simulink model "MBD_week2_prob4"  (R2020b)
settings: Solver=VariableStepAuto  StartTime=0.0  StopTime=0.2  RelTol=1e-3
model workspace (MAT data in the model file):
  J = Simulink.Parameter
  J.Value = 3.2284e-06
  J.DataType = 'auto'
  J.Dimensions = [1 1]
  Ke = Simulink.Parameter
  Ke.Value = 0.0274
  Ke.DataType = 'auto'
  Ke.Dimensions = [1 1]
  Kt = Simulink.Parameter
  Kt.Value = 0.0274
  Kt.DataType = 'auto'
  Kt.Dimensions = [1 1]
  L = Simulink.Parameter
  L.Value = 2.75e-06
  L.DataType = 'auto'
  L.Dimensions = [1 1]
  R = Simulink.Parameter
  R.Value = 4
  R.DataType = 'auto'
  R.Dimensions = [1 1]
  Ts = Simulink.Parameter
  Ts.Value = 0.01
  Ts.DataType = 'auto'
  Ts.Dimensions = [1 1]
  b = Simulink.Parameter
  b.Value = 3.5077e-06
  b.DataType = 'auto'
  b.Dimensions = [1 1]
  kd = Simulink.Parameter
  kd.Value = 50
  kd.DataType = 'auto'
  kd.Dimensions = [1 1]
  ki = Simulink.Parameter
  ki.Value = 22000
  ki.DataType = 'auto'
  ki.Dimensions = [1 1]
  kp = Simulink.Parameter
  kp.Value = 22000
  kp.DataType = 'auto'
  kp.Dimensions = [1 1]
settings Model: Creator=varunraj  LastModifiedBy=varunraj

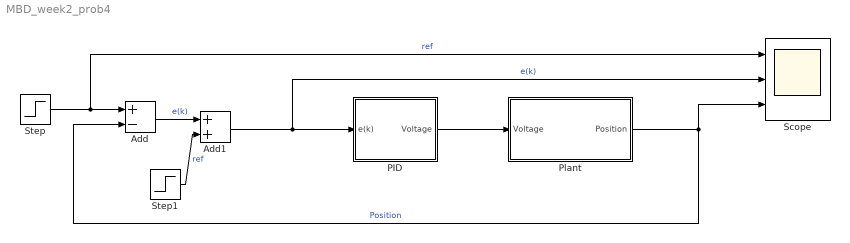
== system MBD_week2_prob4 ==
  Add : Sum  Inputs=+-
  Add1 : Sum
  PID : Subsystem  TreatAsAtomicUnit=on
  Plant : Subsystem  TreatAsAtomicUnit=on
  Scope : Scope  NumInputPorts=3
  Step : Step  Time=0.01  SampleTime=0
  Step1 : Step  Time=0.01  SampleTime=0
  wires:
  Step/1 -> Scope/1, Add/1  "ref"
  Add/1 -> Add1/1  "e(k)"
  Step1/1 -> Add1/2  "ref"
  Add1/1 -> Scope/2, PID/1(e(k))  "e(k)"
  PID/1(Voltage) -> Plant/1(Voltage)
  Plant/1(Position) -> Add/2, Scope/3  "Position"

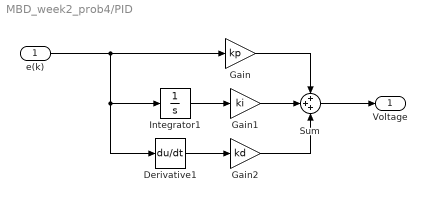
== system MBD_week2_prob4/PID ==
  e(k) : Inport  OutDataTypeStr=double  PortDimensions=1  SampleTime=0
  Derivative1 : Derivative
  Gain : Gain  Gain=kp
  Gain1 : Gain  Gain=ki
  Gain2 : Gain  Gain=kd
  Integrator1 : Integrator
  Sum : Sum  Inputs=+++
  Voltage : Outport  OutDataTypeStr=double  PortDimensions=1  SampleTime=0
  wires:
  Gain/1 -> Sum/1
  Sum/1 -> Voltage/1
  Derivative1/1 -> Gain2/1
  Gain2/1 -> Sum/3
  e(k)/1 -> Gain/1, Integrator1/1, Derivative1/1
  Gain1/1 -> Sum/2
  Integrator1/1 -> Gain1/1

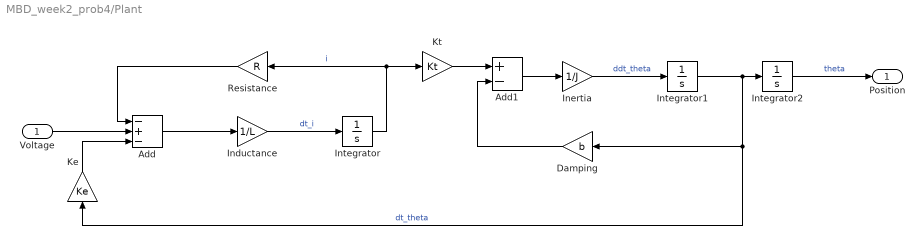
== system MBD_week2_prob4/Plant ==
  Voltage : Inport
  Add : Sum  Inputs=-+-
  Add1 : Sum  Inputs=+-
  Damping : Gain  Gain=b
  Inductance : Gain  Gain=1/L
  Inertia : Gain  Gain=1/J
  Integrator : Integrator
  Integrator1 : Integrator
  Integrator2 : Integrator
  Ke : Gain  Gain=Ke
  Kt : Gain  Gain=Kt
  Resistance : Gain  Gain=R
  Position : Outport
  wires:
  Add/1 -> Inductance/1
  Voltage/1 -> Add/2
  Kt/1 -> Add1/1
  Integrator1/1 -> Ke/1, Damping/1, Integrator2/1  "dt_theta"
  Integrator/1 -> Resistance/1, Kt/1  "i"
  Ke/1 -> Add/3
  Inertia/1 -> Integrator1/1  "ddt_theta"
  Resistance/1 -> Add/1
  Integrator2/1 -> Position/1  "theta"
  Add1/1 -> Inertia/1
  Inductance/1 -> Integrator/1  "dt_i"
  Damping/1 -> Add1/2
